simulink model "MCU_vectorControl_with_fieldWeakening_dsPIC33CK_LVMC_FW_Hurst"  (R2023b)
settings: Solver=FixedStepDiscrete  StartTime=0.0  StopTime=10.0  FixedStep=50e-6  RelTol=1e-3  EnableMultiTasking=on
values from neighbouring files (symbols this model uses):
  w = median(A([end-100:end],9))    [DataVisu.m]
undefined symbols (not defined in the file or in its folder): A0, A4, AN0, AN1, B0, B2, C12, C13, C14, C7, control, D11, D12, D13, D14, D5, D6, D7, DiscIntNeverNeededParam, inverter, Max, MaxPer, model, ms, NumBits1, NumBits2, P20, P32, P55, P60, P61, P62, P69, P70, P71, P75, P76, P77, P78, Pin, pmsm, PosRange1, PosRange2, PWM1max, Resol, s, Slope1, Slope2, us
libraries: simulink x45, MCHP_Blockset x22
(part 4 of 4)

== system MCU_vectorControl_with_fieldWeakening_dsPIC33CK_LVMC_FW_Hurst/Selector/Mode Toggle ==
  state : Inport
  Bitwise Operator : simulink/Logic and Bit Operations/Bitwise Operator  logicop=AND  UseBitMask=on  BitMask=1  BitMaskRealWorld=Stored Integer
  Change when button is pressed : simulink/Logic and Bit Operations/Detect Decrease  vinit=0.0  OutDataTypeStr=uint8
  Sum : Sum  OutDataTypeStr=uint16  AccumDataTypeStr=uint16
  Unit Delay : UnitDelay  SampleTime=-1  HasFrameUpgradeWarning=on
  Mode : Outport  PortDimensions=1  VectorParamsAs1DForOutWhenUnconnected=off
  wires:
  state/1 -> Change when button is pressed/1
  Sum/1 -> Bitwise Operator/1
  Unit Delay/1 -> Sum/2
  Bitwise Operator/1 -> Unit Delay/1, Mode/1
  Change when button is pressed/1 -> Sum/1

== system MCU_vectorControl_with_fieldWeakening_dsPIC33CK_LVMC_FW_Hurst/Selector/On//Off Toggle ==
  in : Inport
  Change when button is pressed : simulink/Logic and Bit Operations/Detect Decrease  vinit=0.0  OutDataTypeStr=uint8
  Logical Operator : Logic  Operator=XOR  AllPortsSameDT=off  OutDataTypeStr=boolean
  Unit Delay : UnitDelay  SampleTime=-1  HasFrameUpgradeWarning=on
  Toggle : Outport  VectorParamsAs1DForOutWhenUnconnected=off
  wires:
  Logical Operator/1 -> Toggle/1, Unit Delay/1  "Toggle"
  in/1 -> Change when button is pressed/1
  Change when button is pressed/1 -> Logical Operator/1
  Unit Delay/1 -> Logical Operator/2

== system MCU_vectorControl_with_fieldWeakening_dsPIC33CK_LVMC_FW_Hurst/Selector/Subsystem ==
  Enable : EnablePort  StatesWhenEnabling=reset
  Constant : Constant  Value=model.omMax/60  OutMax=[20]  OutDataTypeStr=fixdt(1,16)  SampleTime=0.01
  Discrete-Time Integrator : DiscreteIntegrator  SampleTime=-1  OutMax=[1000]  OutDataTypeStr=fixdt(1,16)  SaturateOnIntegerOverflow=on  ICPrevOutput=DiscIntNeverNeededParam  ICPrevScaledInput=DiscIntNeverNeededParam
  Saturation : Saturate  UpperLimit=1000  LowerLimit=100
  Out1 : Outport
  wires:
  Discrete-Time Integrator/1 -> Saturation/1
  Constant/1 -> Discrete-Time Integrator/1
  Saturation/1 -> Out1/1

== system MCU_vectorControl_with_fieldWeakening_dsPIC33CK_LVMC_FW_Hurst/BOARD dsPIC33CK LVMC/Center & sign reversal/Downsample Averaged 2000 samples remove bias ==
  note: DownSample & Average by changing data scaling
  In1 : Inport
  Enable : EnablePort
  Compare To Constant : simulink/Logic and Bit Operations/Compare To Constant  relop===  const=1  OutDataTypeStr=boolean
  Counter Limited : simulink/Sources/Counter Limited  uplimit=DownSample-1  tsamp=-1
  Data Type Duplicate : DataTypeDuplicate
  Data Type Propagation : simulink/Signal Attributes/Data Type Propagation  PropDataType=fixdt(1, 16)  IfRefDouble=double  IfRefSingle=single  IsSigned=IsSigned1 or IsSigned2  NumBitsBase=NumBits1+NumBits2  NumBitsMult=1  NumBitsAdd=0  NumBitsAllowFinal=1:128  PropScaling=2^-10  ValuesUsedBestPrec=[5 -7]  SlopeBase=Slope1  SlopeMult=1  SlopeAdd=0  BiasBase=Bias1  BiasMult=1  BiasAdd=0
  Data Type Propagation1 : simulink/Signal Attributes/Data Type Propagation  PropDataType=fixdt(1, 16)  IfRefDouble=double  IfRefSingle=single  IsSigned=IsSigned1 or IsSigned2  NumBitsBase=NumBits1+NumBits2  NumBitsMult=1  NumBitsAdd=0  NumBitsAllowFinal=1:128  PropScaling=2^-10  ValuesUsedBestPrec=[5 -7]  SlopeBase=PosRange1  SlopeMult=1  SlopeAdd=0  BiasBase=Bias1  BiasMult=1  BiasAdd=0
  Discrete-Time Integrator : DiscreteIntegrator  IntegratorMethod=Accumulation: Backward Euler  gainval=1  ExternalReset=sampled level  SampleTime=-1  OutDataTypeStr=Inherit: Inherit via back propagation  ICPrevOutput=DiscIntNeverNeededParam  ICPrevScaledInput=DiscIntNeverNeededParam
  Gain : Gain  Gain=1/DownSample  OutDataTypeStr=Inherit: Inherit via back propagation  RndMeth=Round
  Gain1 : Gain  Gain=1/DownSample  OutDataTypeStr=Inherit: Inherit via back propagation
  Rate Transition1 : RateTransition  OutPortSampleTimeOpt=Multiple of input port sample time  OutPortSampleTimeMultiple=DownSample  OutPortSampleTime=DownSample
  Rate Transition3 : RateTransition  OutPortSampleTimeOpt=Multiple of input port sample time  OutPortSampleTimeMultiple=DownSample  OutPortSampleTime=DownSample
  Terminator : Terminator
  Out1 : Outport  VectorParamsAs1DForOutWhenUnconnected=off
  wires:
  Rate Transition3/1 -> Gain1/1, Gain/1
  In1/1 -> Rate Transition1/1, Discrete-Time Integrator/1, Data Type Propagation/2, Data Type Propagation/1
  Compare To Constant/1 -> Discrete-Time Integrator/2
  Discrete-Time Integrator/1 -> Data Type Propagation/3, Rate Transition3/1
  Counter Limited/1 -> Compare To Constant/1
  Gain/1 -> Data Type Duplicate/2, Out1/1
  Rate Transition1/1 -> Data Type Propagation1/2, Data Type Propagation1/1, Data Type Duplicate/1
  Gain1/1 -> Terminator/1, Data Type Propagation1/3

== system MCU_vectorControl_with_fieldWeakening_dsPIC33CK_LVMC_FW_Hurst/BOARD dsPIC33CK LVMC/Timing Analysis/Downsample Averaged2 ==
  note: DownSample & Average by changing data scaling
  In1 : Inport
  Compare To Constant : simulink/Logic and Bit Operations/Compare To Constant  relop===  const=1  OutDataTypeStr=boolean
  Counter Limited : simulink/Sources/Counter Limited  uplimit=DownSample-1  tsamp=-1
  Data Type Duplicate : DataTypeDuplicate
  Data Type Propagation : simulink/Signal Attributes/Data Type Propagation  PropDataType=fixdt(1, 16)  IfRefDouble=double  IfRefSingle=single  IsSigned=IsSigned1 or IsSigned2  NumBitsBase=NumBits1+NumBits2  NumBitsMult=1  NumBitsAdd=0  NumBitsAllowFinal=1:128  PropScaling=2^-10  ValuesUsedBestPrec=[5 -7]  SlopeBase=Slope1  SlopeMult=1  SlopeAdd=0  BiasBase=Bias1  BiasMult=1  BiasAdd=0
  Data Type Propagation1 : simulink/Signal Attributes/Data Type Propagation  PropDataType=fixdt(1, 16)  IfRefDouble=double  IfRefSingle=single  IsSigned=IsSigned1 or IsSigned2  NumBitsBase=NumBits1+NumBits2  NumBitsMult=1  NumBitsAdd=0  NumBitsAllowFinal=1:128  PropScaling=2^-10  ValuesUsedBestPrec=[5 -7]  SlopeBase=PosRange1  SlopeMult=1  SlopeAdd=0  BiasBase=Bias1  BiasMult=1  BiasAdd=0
  Discrete-Time Integrator : DiscreteIntegrator  IntegratorMethod=Accumulation: Backward Euler  gainval=1  ExternalReset=sampled level  SampleTime=-1  OutDataTypeStr=Inherit: Inherit via back propagation  ICPrevOutput=DiscIntNeverNeededParam  ICPrevScaledInput=DiscIntNeverNeededParam
  Gain : Gain  Gain=1/DownSample  OutDataTypeStr=Inherit: Inherit via back propagation
  Gain1 : Gain  Gain=1/DownSample  OutDataTypeStr=Inherit: Inherit via back propagation
  Rate Transition1 : RateTransition  Deterministic=off  OutPortSampleTime=[InputSampleTime * DownSample]
  Rate Transition3 : RateTransition  OutPortSampleTime=[InputSampleTime * DownSample]
  Terminator : Terminator
  Out1 : Outport  VectorParamsAs1DForOutWhenUnconnected=off
  wires:
  Gain1/1 -> Terminator/1, Data Type Propagation1/3
  Rate Transition1/1 -> Data Type Duplicate/1, Data Type Propagation1/1, Data Type Propagation1/2
  Gain/1 -> Out1/1, Data Type Duplicate/2
  Counter Limited/1 -> Compare To Constant/1
  Discrete-Time Integrator/1 -> Rate Transition3/1, Data Type Propagation/3
  Compare To Constant/1 -> Discrete-Time Integrator/2
  In1/1 -> Data Type Propagation/1, Data Type Propagation/2, Rate Transition1/1, Discrete-Time Integrator/1
  Rate Transition3/1 -> Gain/1, Gain1/1

== system MCU_vectorControl_with_fieldWeakening_dsPIC33CK_LVMC_FW_Hurst/Control law/Speed control/Current Control ==
  idqref : Inport
  idq : Inport  Port=2
  Data Type Duplicate : DataTypeDuplicate  Commented=on  NumInputPorts=3
  Data Type Propagation : simulink/Signal Attributes/Data Type Propagation  Commented=on  PropDataType=fixdt(1, 16)  IfRefDouble=double  IfRefSingle=single  IsSigned=IsSigned1 or IsSigned2  NumBitsBase=max([NumBits1 NumBits2])  NumBitsMult=1  NumBitsAdd=0  NumBitsAllowFinal=1:128  PropScaling=2^-(15-ceil(log2(2*inverter.iMax)))  ValuesUsedBestPrec=[5 -7]  SlopeBase=max([PosRange1 PosRange2])  SlopeMult=2  SlopeAdd=0  BiasBase=Bias1  BiasMult=1  BiasAdd=0
  Data Type Propagation2 : simulink/Signal Attributes/Data Type Propagation  PropDataType=fixdt(1, 16)  IfRefDouble=double  IfRefSingle=single  IsSigned=TRUE  NumBitsBase=max([NumBits1 NumBits2])  NumBitsMult=1  NumBitsAdd=0  NumBitsAllowFinal=[1:128]  PropScaling=2^-(15-ceil(log2(inverter.vDC/sqrt(3))))  ValuesUsedBestPrec=[100 -100]  SlopeBase=max([PosRange1 PosRange2])  SlopeMult=abs(control.kE(2))  SlopeAdd=0  BiasBase=Bias1  BiasMult=1  BiasAdd=0
  Gain : Gain  Gain=control.kE(2)  OutDataTypeStr=Inherit: Inherit via back propagation  SaturateOnIntegerOverflow=on
  Gain1 : Gain  Gain=control.kE(1)  OutDataTypeStr=Inherit: Inherit via back propagation  SaturateOnIntegerOverflow=on
  Integrator : Subsystem
  Sum : Sum  Inputs=|--  OutDataTypeStr=Inherit: Inherit via back propagation  SaturateOnIntegerOverflow=on
  Sum3 : Sum  Inputs=|+-  OutDataTypeStr=Inherit: Inherit via back propagation  SaturateOnIntegerOverflow=on
  v : Outport  VectorParamsAs1DForOutWhenUnconnected=off
  wires:
  Sum/1 -> v/1, Data Type Duplicate/1
  idqref/1 -> Sum3/1, Data Type Propagation/1
  idq/1 -> Sum3/2, Gain1/1, Data Type Propagation/2
  Gain1/1 -> Sum/2, Data Type Duplicate/3
  Integrator/1(Out1) -> Sum/1
  Gain/1 -> Data Type Propagation2/3, Integrator/1(In1)
  Sum3/1 -> Data Type Propagation2/2, Data Type Propagation2/1, Gain/1, Data Type Propagation/3

== system MCU_vectorControl_with_fieldWeakening_dsPIC33CK_LVMC_FW_Hurst/Control law/Speed control/Mechanical Control ==
  omref : Inport
  om : Inport  Port=2
  isat : Inport  Port=3
  Clamping circuit : Subsystem
  Constant : Constant  Value=0  OutMax=model.iMax  OutDataTypeStr=fixdt(1,16)
  Data Type Duplicate1 : DataTypeDuplicate
  Data Type Propagation : simulink/Signal Attributes/Data Type Propagation  PropDataType=fixdt(1, 16)  IfRefDouble=double  IfRefSingle=single  IsSigned=IsSigned1 or IsSigned2  NumBitsBase=max([NumBits1 NumBits2])  NumBitsMult=1  NumBitsAdd=0  NumBitsAllowFinal=1:128  PropScaling=2^-(15-ceil(log2(2*pmsm.omMax)))  ValuesUsedBestPrec=[5 -7]  SlopeBase=max([PosRange1 PosRange2])  SlopeMult=2  SlopeAdd=0  BiasBase=Bias1  BiasMult=1  BiasAdd=0
  Delay : Delay  DelayLength=1
  Gain : Gain  Gain=control.kM(2)  OutDataTypeStr=Inherit: Inherit via back propagation  SaturateOnIntegerOverflow=on
  Gain1 : Gain  Gain=control.kM(1)  OutMax=model.iMax  OutDataTypeStr=fixdt(1,16)  SaturateOnIntegerOverflow=on
  Integrator : Subsystem
  Saturation Dynamic : simulink/Discontinuities/Saturation Dynamic  OutMin=[]  OutMax=[]  OutDataTypeStr=Inherit: Same as second input  OutDataType=fixdt(1, 16)  OutScaling=2^-10  DoSatur=off
  Sum : Sum  Inputs=|--  OutMax=model.iMax  OutDataTypeStr=fixdt(1,16)  SaturateOnIntegerOverflow=on
  Sum1 : Sum  Inputs=|+-  OutDataTypeStr=Inherit: Inherit via back propagation
  Sum2 : Sum  Inputs=|-+  SaturateOnIntegerOverflow=on  OutDataTypeStr=Inherit: Same as first input
  iqref : Outport  VectorParamsAs1DForOutWhenUnconnected=off
  wires:
  Saturation Dynamic/1 -> Sum2/1, iqref/1
  Sum/1 -> Sum2/2, Saturation Dynamic/2
  Gain/1 -> Sum/1
  om/1 -> Sum1/2, Gain1/1, Data Type Propagation/2, Data Type Duplicate1/2
  Sum1/1 -> Integrator/1(In1), Clamping circuit/2(preIntegrator), Data Type Propagation/3
  omref/1 -> Sum1/1, Data Type Propagation/1, Data Type Duplicate1/1
  Clamping circuit/1(Clamp) -> Integrator/Enable
  Sum2/1 -> Clamping circuit/1(Saturation)
  Integrator/1(Out1) -> Gain/1
  Gain1/1 -> Sum/2
  isat/1 -> Delay/1
  Delay/1 -> Saturation Dynamic/1
  Constant/1 -> Saturation Dynamic/3

== system MCU_vectorControl_with_fieldWeakening_dsPIC33CK_LVMC_FW_Hurst/Control law/Speed control/Subsystem2 ==
  om : Inport
  iref : Inport  Port=2
  Imax : Inport  Port=3
  Subsystem6 : Subsystem
  decision1 : Subsystem
  idq : Outport
  isat : Outport  Port=2
  wires:
  Imax/1 -> decision1/1(Imax), Subsystem6/1(Imax)
  Subsystem6/7(delta) -> decision1/9(delta)
  decision1/2(isat) -> isat/1
  Subsystem6/6(c(w)) -> decision1/8(c(w))
  Subsystem6/5(b(w)) -> decision1/7(b(w))
  Subsystem6/4(a(w)) -> decision1/6(a(w))
  Subsystem6/1(i1(w)) -> decision1/3(i1(w))
  Subsystem6/3(i4(w)) -> decision1/5(i3(w))
  Subsystem6/2(i2(w)) -> decision1/4(i2(w))
  decision1/1(idq) -> idq/1
  iref/1 -> decision1/2(iqref)
  om/1 -> Subsystem6/2(om)

== system MCU_vectorControl_with_fieldWeakening_dsPIC33CK_LVMC_FW_Hurst/Control law/Speed control/Current Control/Integrator ==
  In1 : Inport
  Data Type Propagation : simulink/Signal Attributes/Data Type Propagation  PropDataType=fixdt(1, 16)  IfRefDouble=single  IfRefSingle=single  IsSigned=IsSigned1 or IsSigned2  NumBitsBase=NumBits1+NumBits2  NumBitsMult=1  NumBitsAdd=0  NumBitsAllowFinal=1:128  PropScalingMode=Specify via dialog  PropScaling=2^-23  ValuesUsedBestPrec=[5 -7]  SlopeBase=min([Slope1 Slope2])  SlopeMult=1  SlopeAdd=0  BiasBase=Bias1  BiasMult=1  BiasAdd=0
  Discrete-Time Integrator : DiscreteIntegrator  SampleTime=-1  OutDataTypeStr=Inherit: Inherit via back propagation  SaturateOnIntegerOverflow=on  ICPrevOutput=DiscIntNeverNeededParam  ICPrevScaledInput=DiscIntNeverNeededParam
  Out1 : Outport  VectorParamsAs1DForOutWhenUnconnected=off
  wires:
  Discrete-Time Integrator/1 -> Out1/1, Data Type Propagation/3
  In1/1 -> Data Type Propagation/1, Data Type Propagation/2, Discrete-Time Integrator/1

== system MCU_vectorControl_with_fieldWeakening_dsPIC33CK_LVMC_FW_Hurst/Control law/Speed control/Mechanical Control/Clamping circuit ==
  note: The clamping enable or disable the integral action.
  Saturation : Inport  DisableCoverage=on
  preIntegrator : Inport  DisableCoverage=on  Port=2
  Compare To Zero1 : simulink/Logic and Bit Operations/Compare To Zero  relop=<=  OutDataTypeStr=boolean
  Delay : Delay  DelayLength=1  InitialCondition=0
  Multiply : Product  SaturateOnIntegerOverflow=on  OutDataTypeStr=Inherit: Same as first input
  Clamp : Outport  DisableCoverage=on  VectorParamsAs1DForOutWhenUnconnected=off
  wires:
  Delay/1 -> Multiply/1
  Saturation/1 -> Delay/1
  Multiply/1 -> Compare To Zero1/1
  preIntegrator/1 -> Multiply/2
  Compare To Zero1/1 -> Clamp/1

== system MCU_vectorControl_with_fieldWeakening_dsPIC33CK_LVMC_FW_Hurst/Control law/Speed control/Mechanical Control/Integrator ==
  In1 : Inport
  Enable : EnablePort
  Discrete-Time Integrator : DiscreteIntegrator  SampleTime=-1  OutDataTypeStr=fixdt(1,32,20)  SaturateOnIntegerOverflow=on  ICPrevOutput=DiscIntNeverNeededParam  ICPrevScaledInput=DiscIntNeverNeededParam
  Out1 : Outport  VectorParamsAs1DForOutWhenUnconnected=off
  wires:
  In1/1 -> Discrete-Time Integrator/1
  Discrete-Time Integrator/1 -> Out1/1

== system MCU_vectorControl_with_fieldWeakening_dsPIC33CK_LVMC_FW_Hurst/Control law/Speed control/Subsystem2/Subsystem6 ==
  Imax : Inport
  om : Inport  Port=2
  Compare To Constant : simulink/Logic and Bit Operations/Compare To Constant  relop=>  const=model.omBase  OutDataTypeStr=boolean
  Constant : Constant  Value=0  OutMax=model.iMax  OutDataTypeStr=fixdt(1,16)
  Contraints (9) fix : Subsystem
  Subsystem3 : Subsystem
  Subsystem4 : Subsystem
  Subsystem5 : Subsystem
  Switch : Switch  Criteria=u2 > Threshold  SaturateOnIntegerOverflow=off  InputSameDT=off
  i1(w) : Outport
  i2(w) : Outport  Port=2
  i4(w) : Outport  Port=3
  a(w) : Outport  Port=4
  b(w) : Outport  Port=5
  c(w) : Outport  Port=6
  delta : Outport  Port=7
  wires:
  Subsystem4/2(delta) -> delta/1
  Constant/1 -> Switch/3
  Subsystem5/1(i4(w)) -> i4(w)/1
  Switch/1 -> i2(w)/1
  Subsystem3/1(i1(w)) -> i1(w)/1
  Contraints (9) fix/1(a(w)) -> a(w)/1, Subsystem3/1(a(w)), Subsystem4/1(a(w))
  Contraints (9) fix/2(b(w)) -> b(w)/1, Subsystem3/2(b(w)), Subsystem4/2(b(w)), Subsystem5/1(b(w))
  Subsystem4/1(i2(w)) -> Switch/1
  Compare To Constant/1 -> Switch/2, Subsystem4/Enable
  Contraints (9) fix/3(c(w)) -> c(w)/1, Subsystem3/3(c(w)), Subsystem4/3(c(w)), Subsystem5/2(c(w))
  Imax/1 -> Subsystem4/4(Imax)
  om/1 -> Compare To Constant/1, Contraints (9) fix/1(om)

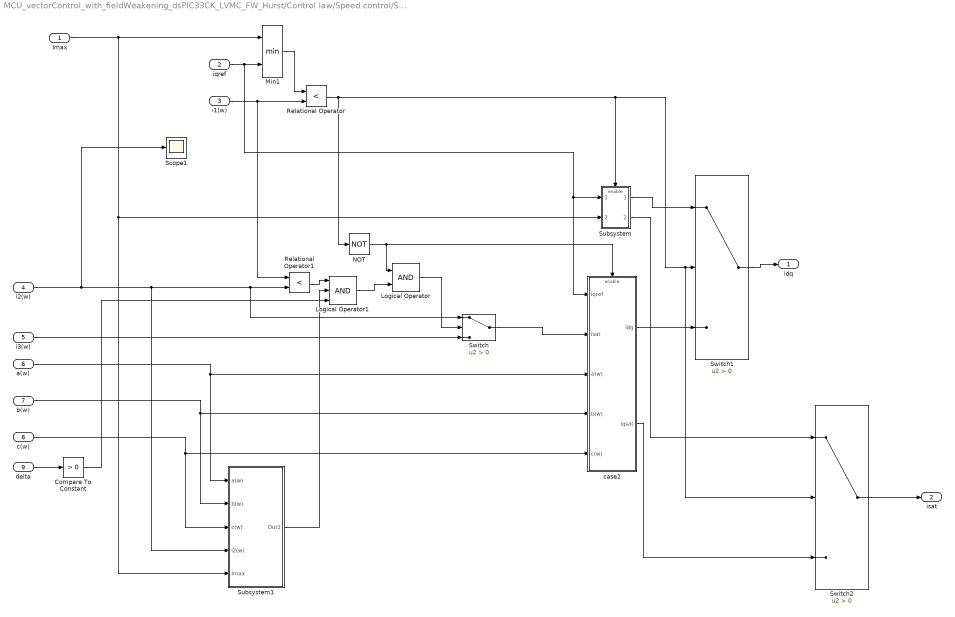
== system MCU_vectorControl_with_fieldWeakening_dsPIC33CK_LVMC_FW_Hurst/Control law/Speed control/Subsystem2/decision1 ==
  Imax : Inport
  iqref : Inport  Port=2
  i1(w) : Inport  Port=3
  i2(w) : Inport  Port=4
  i3(w) : Inport  Port=5
  a(w) : Inport  Port=6
  b(w) : Inport  Port=7
  c(w) : Inport  Port=8
  delta : Inport  Port=9
  Compare To Constant : simulink/Logic and Bit Operations/Compare To Constant  relop=>  const=0  OutDataTypeStr=boolean
  Logical Operator : Logic  AllPortsSameDT=off  OutDataTypeStr=boolean
  Logical Operator1 : Logic  Inputs=3  AllPortsSameDT=off  OutDataTypeStr=boolean
  Min1 : MinMax  Inputs=2
  NOT : Logic  Operator=NOT  IconShape=distinctive  AllPortsSameDT=off  OutDataTypeStr=boolean
  Relational Operator : RelationalOperator  Operator=<  OutDataTypeStr=boolean  RndMeth=Simplest  InputSameDT=off
  Relational Operator1 : RelationalOperator  Operator=<  OutDataTypeStr=boolean  RndMeth=Simplest  InputSameDT=off
  Scope1 : Scope
  Subsystem : Subsystem
  Subsystem1 : Subsystem
  Switch : Switch  Criteria=u2 > Threshold  SaturateOnIntegerOverflow=off  InputSameDT=off
  Switch1 : Switch  Criteria=u2 > Threshold  SaturateOnIntegerOverflow=off  InputSameDT=off
  Switch2 : Switch  Criteria=u2 > Threshold  SaturateOnIntegerOverflow=off  InputSameDT=off
  case2 : Subsystem
  idq : Outport
  isat : Outport  Port=2
  wires:
  Switch2/1 -> isat/1
  case2/2(iqsat) -> Switch2/3
  Subsystem/2(iqsat) -> Switch2/1
  Compare To Constant/1 -> Logical Operator1/3
  delta/1 -> Compare To Constant/1
  Switch/1 -> case2/2(isat)
  i2(w)/1 -> Switch/1, Relational Operator1/2, Subsystem1/4(i2(w)), Scope1/1
  Logical Operator1/1 -> Logical Operator/2
  Relational Operator1/1 -> Logical Operator1/1
  Imax/1 -> Min1/1, Subsystem1/5(Imax), Subsystem/2(iMax)
  Subsystem1/1(Out1) -> Logical Operator1/2
  Min1/1 -> Relational Operator/1
  Relational Operator/1 -> NOT/1, Subsystem/Enable, Switch1/2, Switch2/2
  case2/1(idq) -> Switch1/3
  Switch1/1 -> idq/1
  i1(w)/1 -> Relational Operator1/1, Relational Operator/2
  Subsystem/1(idq) -> Switch1/1
  NOT/1 -> Logical Operator/1, case2/Enable
  Logical Operator/1 -> Switch/2
  iqref/1 -> Min1/2, case2/1(iqref), Subsystem/1(iref)
  i3(w)/1 -> Switch/3
  a(w)/1 -> case2/3(a(w)), Subsystem1/1(a(w))
  b(w)/1 -> case2/4(b(w)), Subsystem1/2(b(w))
  c(w)/1 -> case2/5(c(w)), Subsystem1/3(c(w))

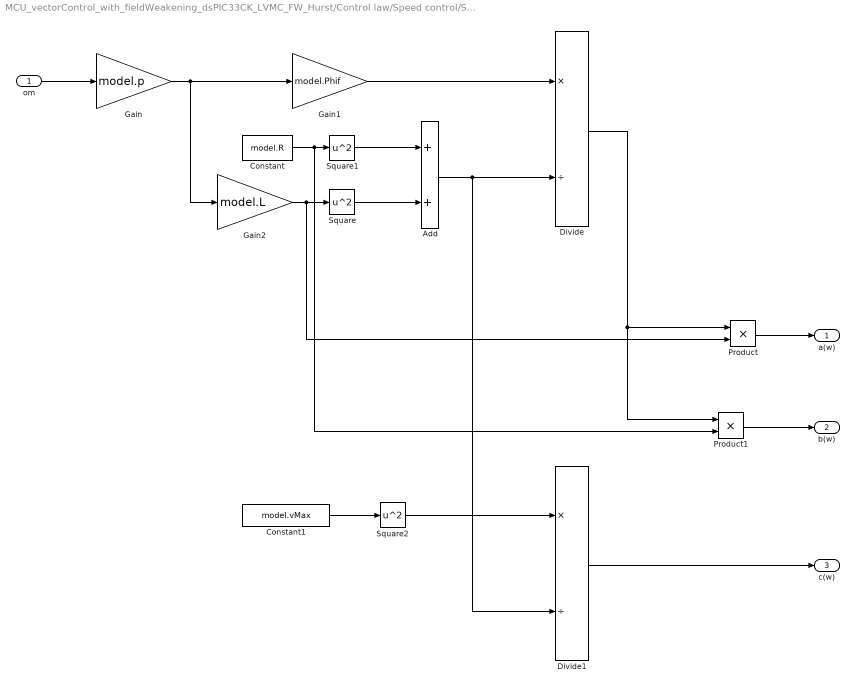
== system MCU_vectorControl_with_fieldWeakening_dsPIC33CK_LVMC_FW_Hurst/Control law/Speed control/Subsystem2/Subsystem6/Contraints (9) fix ==
  om : Inport
  Add : Sum  OutMax=(model.R.^2+(model.p*model.omMax*model.L).^2)  OutDataTypeStr=fixdt(0,16)  SaturateOnIntegerOverflow=on
  Constant : Constant  Value=model.R  OutMax=model.R  OutDataTypeStr=fixdt(0,16)
  Constant1 : Constant  Value=model.vMax  OutMax=model.vMax  OutDataTypeStr=fixdt(0,16)
  Divide : Product  Inputs=*/  OutMax=max((model.p*(0:0.1:model.omMax)*model.Phif./(model.R.^2+(model.p*(0:0.1:model.omMax)*model.L).^2)))  OutDataTypeStr=fixdt(0,16)
  Divide1 : Product  Inputs=*/  OutMax=max((model.vMax*model.vMax./(model.R.^2+(model.p*(0:0.1:model.omMax)*model.L).^2)))  OutDataTypeStr=fixdt(0,16)  SaturateOnIntegerOverflow=on
  Gain : Gain  Gain=model.p  OutMax=model.p*model.omMax  OutDataTypeStr=fixdt(0,16)
  Gain1 : Gain  Gain=model.Phif  OutMax=model.p*model.Phif*model.omMax  OutDataTypeStr=fixdt(0,16)  SaturateOnIntegerOverflow=on
  Gain2 : Gain  Gain=model.L  OutMax=model.L*model.p*model.omMax  OutDataTypeStr=fixdt(0,16)  SaturateOnIntegerOverflow=on
  Product : Product  OutMax=model.L*model.p*model.omMax*max((model.p*(0:0.1:model.omMax)*model.Phif./(model.R.^2+(model.p*(0:0.1:model.omMax)*model.L).^2)))  OutDataTypeStr=fixdt(0,16)  SaturateOnIntegerOverflow=on
  Product1 : Product  OutMax=model.R*max((model.p*(0:0.1:model.omMax)*model.Phif./(model.R.^2+(model.p*(0:0.1:model.omMax)*model.L).^2)))  OutDataTypeStr=fixdt(0,16)  SaturateOnIntegerOverflow=on
  Square : Math  Operator=square  OutMax=(model.L*model.p*model.omMax)^2  OutDataTypeStr=fixdt(0,16)
  Square1 : Math  Operator=square  OutMax=model.R*model.R  OutDataTypeStr=fixdt(0,16)
  Square2 : Math  Operator=square  OutMax=model.vMax*model.vMax  OutDataTypeStr=fixdt(0,16)
  a(w) : Outport
  b(w) : Outport  Port=2
  c(w) : Outport  Port=3
  wires:
  Square2/1 -> Divide1/1
  Divide1/1 -> c(w)/1
  Gain/1 -> Gain1/1, Gain2/1
  Gain2/1 -> Square/1, Product/2
  Add/1 -> Divide/2, Divide1/2
  Divide/1 -> Product/1, Product1/1
  Constant/1 -> Square1/1, Product1/2
  om/1 -> Gain/1
  Square/1 -> Add/2
  Product/1 -> a(w)/1
  Constant1/1 -> Square2/1
  Gain1/1 -> Divide/1
  Square1/1 -> Add/1
  Product1/1 -> b(w)/1

== system MCU_vectorControl_with_fieldWeakening_dsPIC33CK_LVMC_FW_Hurst/Control law/Speed control/Subsystem2/Subsystem6/Subsystem3 ==
  a(w) : Inport
  b(w) : Inport  Port=2
  c(w) : Inport  Port=3
  Add : Sum  Inputs=+-  SaturateOnIntegerOverflow=on  OutDataTypeStr=Inherit: Same as first input
  Add1 : Sum  Inputs=+-  OutMax=model.iMax  OutDataTypeStr=fixdt(1,16)  SaturateOnIntegerOverflow=on
  Constant1 : Constant  Value=0  OutDataTypeStr=int16
  Sqrt : Sqrt
  Square : Math  Operator=square  OutMax=(model.L*model.p*model.omMax*max((model.p*(0:0.1:model.omMax)*model.Phif./(model.R.^2+(model.p*(0:0.1:model.omMax)*model.L).^2)))).^2  OutDataTypeStr=fixdt(0,16)
  Switch2 : Switch  Criteria=u2 > Threshold  SaturateOnIntegerOverflow=off  InputSameDT=off  OutDataTypeStr=Inherit: Same as first input
  Switch3 : Switch  Criteria=u2 > Threshold  SaturateOnIntegerOverflow=off  InputSameDT=off  OutDataTypeStr=Inherit: Same as first input
  i1(w) : Outport
  wires:
  Switch3/1 -> i1(w)/1
  Switch2/1 -> Sqrt/1
  Constant1/1 -> Switch2/3, Switch3/3
  Add/1 -> Switch2/2, Switch3/2, Switch2/1
  Sqrt/1 -> Add1/1
  b(w)/1 -> Add1/2
  c(w)/1 -> Add/1
  a(w)/1 -> Square/1
  Square/1 -> Add/2
  Add1/1 -> Switch3/1

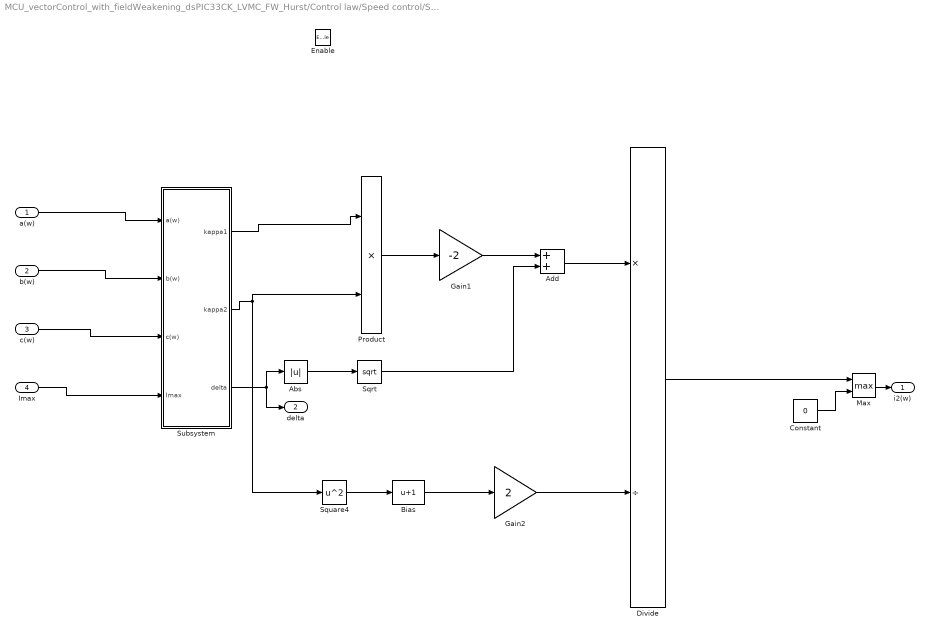
== system MCU_vectorControl_with_fieldWeakening_dsPIC33CK_LVMC_FW_Hurst/Control law/Speed control/Subsystem2/Subsystem6/Subsystem4 ==
  a(w) : Inport
  b(w) : Inport  Port=2
  c(w) : Inport  Port=3
  Imax : Inport  Port=4
  Enable : EnablePort
  Abs : Abs  SaturateOnIntegerOverflow=off
  Add : Sum  OutMax=[2*model.iMax^2]  OutDataTypeStr=fixdt(1,16)
  Bias : Bias  Bias=1  SaturateOnIntegerOverflow=off
  Constant : Constant  Value=0  OutMax=[model.iMax]  OutDataTypeStr=fixdt(1,16)
  Divide : Product  Inputs=*/  OutMax=[model.iMax]  OutDataTypeStr=fixdt(1,16)
  Gain1 : Gain  Gain=-2  OutMax=[model.iMax^2]  OutDataTypeStr=fixdt(1,16)
  Gain2 : Gain  Gain=2  OutMax=[2*model.iMax^2]  OutDataTypeStr=fixdt(1,16)
  Max : MinMax  Function=max  Inputs=2  OutDataTypeStr=Inherit: Same as first input
  Product : Product  OutMax=model.iMax*model.iMax  OutDataTypeStr=fixdt(1,16)
  Sqrt : Sqrt  OutMax=[4*model.iMax^2]  OutDataTypeStr=fixdt(1,16)
  Square4 : Math  Operator=square  OutMax=[model.iMax^2]  OutDataTypeStr=fixdt(1,16)
  Subsystem : Subsystem
  i2(w) : Outport
  delta : Outport  Port=2
  wires:
  a(w)/1 -> Subsystem/1(a(w))
  b(w)/1 -> Subsystem/2(b(w))
  Imax/1 -> Subsystem/4(Imax)
  c(w)/1 -> Subsystem/3(c(w))
  Subsystem/1(kappa1) -> Product/1
  Abs/1 -> Sqrt/1
  Divide/1 -> Max/1
  Add/1 -> Divide/1
  Product/1 -> Gain1/1
  Sqrt/1 -> Add/2
  Gain2/1 -> Divide/2
  Gain1/1 -> Add/1
  Square4/1 -> Bias/1
  Constant/1 -> Max/2
  Bias/1 -> Gain2/1
  Max/1 -> i2(w)/1
  Subsystem/2(kappa2) -> Square4/1, Product/2
  Subsystem/3(delta) -> delta/1, Abs/1

== system MCU_vectorControl_with_fieldWeakening_dsPIC33CK_LVMC_FW_Hurst/Control law/Speed control/Subsystem2/Subsystem6/Subsystem5 ==
  b(w) : Inport
  c(w) : Inport  Port=2
  Add : Sum  Inputs=+-  OutMax=2*model.iMax  OutDataTypeStr=fixdt(0,16)  SaturateOnIntegerOverflow=on
  Sqrt : Sqrt  OutMax=2*model.iMax  OutDataTypeStr=fixdt(0,16)
  i4(w) : Outport
  wires:
  Add/1 -> i4(w)/1
  c(w)/1 -> Sqrt/1
  Sqrt/1 -> Add/1
  b(w)/1 -> Add/2

== system MCU_vectorControl_with_fieldWeakening_dsPIC33CK_LVMC_FW_Hurst/Control law/Speed control/Subsystem2/decision1/Subsystem ==
  iref : Inport
  iMax : Inport  Port=2
  Enable : EnablePort
  Constant : Constant  Value=0  OutMax=model.iMax  OutDataTypeStr=fixdt(1,16)
  Min : MinMax  Inputs=2
  Mux : Mux  Inputs=2
  idq : Outport
  iqsat : Outport  Port=2
  wires:
  iMax/1 -> Min/2, iqsat/1
  Mux/1 -> idq/1
  iref/1 -> Min/1
  Min/1 -> Mux/2
  Constant/1 -> Mux/1

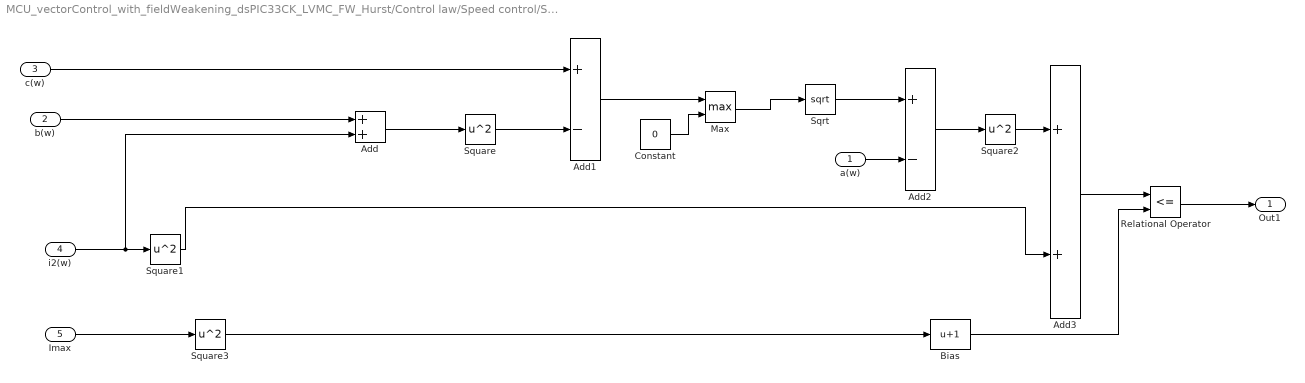
== system MCU_vectorControl_with_fieldWeakening_dsPIC33CK_LVMC_FW_Hurst/Control law/Speed control/Subsystem2/decision1/Subsystem1 ==
  a(w) : Inport
  b(w) : Inport  Port=2
  c(w) : Inport  Port=3
  i2(w) : Inport  Port=4
  Imax : Inport  Port=5
  Add : Sum  OutMax=2*model.iMax  OutDataTypeStr=fixdt(1,16)  SaturateOnIntegerOverflow=on
  Add1 : Sum  Inputs=+-  OutDataTypeStr=fixdt(1,16,6)  AccumDataTypeStr=fixdt(1,32,20)  SaturateOnIntegerOverflow=on
  Add2 : Sum  Inputs=+-  OutMax=3*model.iMax  OutDataTypeStr=fixdt(1,16)  AccumDataTypeStr=fixdt(1,32,20)  SaturateOnIntegerOverflow=on
  Add3 : Sum  OutMax=4*model.iMax*model.iMax  OutDataTypeStr=fixdt(1,16)  AccumDataTypeStr=fixdt(1,32,20)  SaturateOnIntegerOverflow=on
  Bias : Bias  Bias=1
  Constant : Constant  Value=0  OutDataTypeStr=int16
  Max : MinMax  Function=max  Inputs=2  SaturateOnIntegerOverflow=on  OutDataTypeStr=Inherit: Same as first input
  Relational Operator : RelationalOperator  Operator=<=  OutDataTypeStr=boolean  RndMeth=Simplest  InputSameDT=off
  Sqrt : Sqrt  OutMax=3*model.iMax  OutDataTypeStr=fixdt(1,16)
  Square : Math  Operator=square  OutDataTypeStr=fixdt(1,16,6)
  Square1 : Math  Operator=square  OutMax=model.iMax*model.iMax  OutDataTypeStr=fixdt(1,16)
  Square2 : Math  Operator=square  OutDataTypeStr=fixdt(1,16,6)
  Square3 : Math  Operator=square  OutMax=9*model.iMax*model.iMax  OutDataTypeStr=fixdt(1,16)
  Out1 : Outport
  wires:
  b(w)/1 -> Add/1
  c(w)/1 -> Add1/1
  i2(w)/1 -> Square1/1, Add/2
  Imax/1 -> Square3/1
  Max/1 -> Sqrt/1
  Constant/1 -> Max/2
  Add1/1 -> Max/1
  Relational Operator/1 -> Out1/1
  Bias/1 -> Relational Operator/2
  Square3/1 -> Bias/1
  Add3/1 -> Relational Operator/1
  Square2/1 -> Add3/1
  a(w)/1 -> Add2/2
  Square1/1 -> Add3/2
  Add2/1 -> Square2/1
  Square/1 -> Add1/2
  Sqrt/1 -> Add2/1
  Add/1 -> Square/1

== system MCU_vectorControl_with_fieldWeakening_dsPIC33CK_LVMC_FW_Hurst/Control law/Speed control/Subsystem2/decision1/case2 ==
  iqref : Inport
  isat : Inport  Port=2
  a(w) : Inport  Port=3
  b(w) : Inport  Port=4
  c(w) : Inport  Port=5
  Enable : EnablePort
  Add : Sum  OutMax=2*model.iMax  OutDataTypeStr=fixdt(0,16)  SaturateOnIntegerOverflow=on
  Add1 : Sum  Inputs=+-  OutMax=9*model.iMax*model.iMax  OutDataTypeStr=fixdt(1,16)  AccumDataTypeStr=fixdt(1,32,20)  SaturateOnIntegerOverflow=on
  Add2 : Sum  Inputs=+-  OutMax=model.iMax  OutDataTypeStr=fixdt(1,16)  AccumDataTypeStr=fixdt(1,32,20)  SaturateOnIntegerOverflow=on
  Constant : Constant  Value=0  OutDataTypeStr=int16
  Max : MinMax  Function=max  Inputs=2  SaturateOnIntegerOverflow=on  OutDataTypeStr=Inherit: Same as first input
  Min1 : MinMax  Inputs=2  SaturateOnIntegerOverflow=on  OutDataTypeStr=Inherit: Same as first input
  Mux : Mux  Inputs=2
  Sqrt : Sqrt  OutMax=model.iMax  OutDataTypeStr=fixdt(1,16)
  Square : Math  Operator=square  OutMax=3*model.iMax*model.iMax  OutDataTypeStr=fixdt(0,16)
  idq : Outport
  iqsat : Outport  Port=2
  wires:
  c(w)/1 -> Add1/1
  b(w)/1 -> Add/1
  iqref/1 -> Min1/1
  isat/1 -> Min1/2, iqsat/1
  Constant/1 -> Max/2
  Max/1 -> Sqrt/1
  Min1/1 -> Mux/2, Add/2
  Add/1 -> Square/1
  Square/1 -> Add1/2
  Add1/1 -> Max/1
  Sqrt/1 -> Add2/1
  a(w)/1 -> Add2/2
  Mux/1 -> idq/1
  Add2/1 -> Mux/1

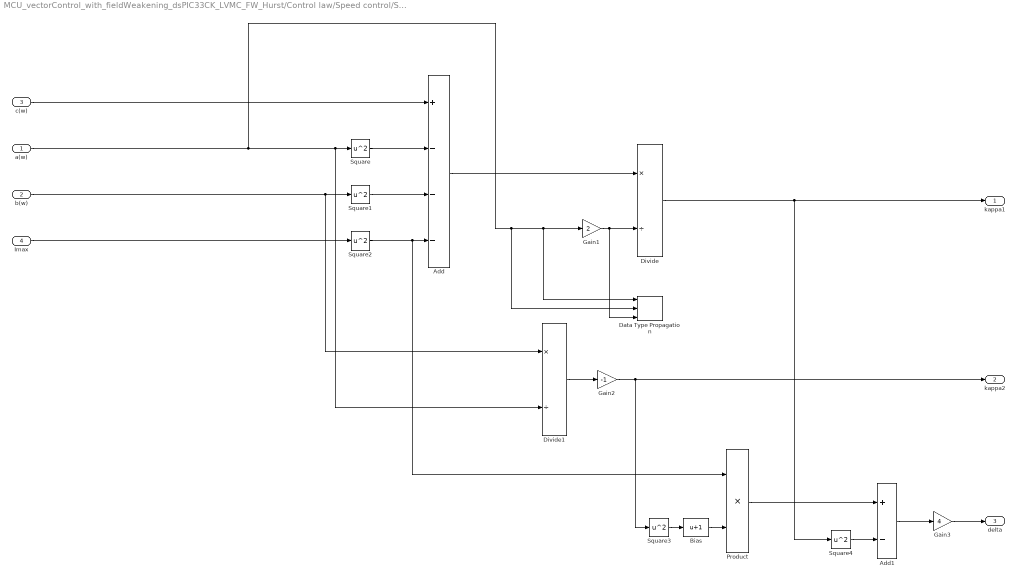
== system MCU_vectorControl_with_fieldWeakening_dsPIC33CK_LVMC_FW_Hurst/Control law/Speed control/Subsystem2/Subsystem6/Subsystem4/Subsystem ==
  a(w) : Inport
  b(w) : Inport  Port=2
  c(w) : Inport  Port=3
  Imax : Inport  Port=4
  Add : Sum  Inputs=+---  OutMax=[3*model.iMax*model.iMax]  OutDataTypeStr=fixdt(1,32)  AccumDataTypeStr=fixdt(1,32,20)  SaturateOnIntegerOverflow=on
  Add1 : Sum  Inputs=+-
  Bias : Bias  Bias=1  SaturateOnIntegerOverflow=off
  Data Type Propagation : simulink/Signal Attributes/Data Type Propagation  PropDataType=fixdt(1, 16)  IfRefDouble=double  IfRefSingle=single  IsSigned=IsSigned1 or IsSigned2  NumBitsBase=max([NumBits1 NumBits2])  NumBitsMult=1  NumBitsAdd=0  NumBitsAllowFinal=1:128  PropScaling=2^-10  ValuesUsedBestPrec=[5 -7]  SlopeBase=max([Slope1 Slope2])  SlopeMult=2  SlopeAdd=0  BiasBase=Bias1  BiasMult=1  BiasAdd=0
  Divide : Product  Inputs=*/  OutMax=[2*model.iMax]  OutDataTypeStr=fixdt(1,16)
  Divide1 : Product  Inputs=*/  OutMax=model.iMax  OutDataTypeStr=fixdt(1,16)
  Gain1 : Gain  Gain=2  OutDataTypeStr=Inherit: Inherit via back propagation
  Gain2 : Gain  Gain=-1  OutDataTypeStr=Inherit: Same as input
  Gain3 : Gain  Gain=4  OutMax=[4*model.iMax^3]  OutDataTypeStr=fixdt(1,16)
  Product : Product  OutMax=[model.iMax^3]  OutDataTypeStr=fixdt(1,16)
  Square : Math  Operator=square  OutMax=(model.L*model.p*model.omMax*max((model.p*(0:0.1:model.omMax)*model.Phif./(model.R.^2+(model.p*(0:0.1:model.omMax)*model.L).^2)))).^2  OutDataTypeStr=fixdt(0,16)
  Square1 : Math  Operator=square  OutMax=(model.R*max((model.p*(0:0.1:model.omMax)*model.Phif./(model.R.^2+(model.p*(0:0.1:model.omMax)*model.L).^2))))^2  OutDataTypeStr=fixdt(0,16)
  Square2 : Math  Operator=square  OutMax=model.iMax^2  OutDataTypeStr=fixdt(0,16)
  Square3 : Math  Operator=square
  Square4 : Math  Operator=square  OutMax=[model.iMax^3]  OutDataTypeStr=fixdt(1,16)
  kappa1 : Outport
  kappa2 : Outport  Port=2
  delta : Outport  Port=3
  wires:
  a(w)/1 -> Gain1/1, Data Type Propagation/1, Data Type Propagation/2, Square/1, Divide1/2
  Divide/1 -> kappa1/1, Square4/1
  c(w)/1 -> Add/1
  b(w)/1 -> Divide1/1, Square1/1
  Imax/1 -> Square2/1
  Gain1/1 -> Divide/2, Data Type Propagation/3
  Bias/1 -> Product/2
  Square4/1 -> Add1/2
  Add1/1 -> Gain3/1
  Add/1 -> Divide/1
  Gain3/1 -> delta/1
  Divide1/1 -> Gain2/1
  Square3/1 -> Bias/1
  Product/1 -> Add1/1
  Square2/1 -> Product/1, Add/4
  Gain2/1 -> kappa2/1, Square3/1
  Square/1 -> Add/2
  Square1/1 -> Add/3
